simulink model "TriggeredEnabled_Subsystem"  (R2017b)
settings: Solver=FixedStepDiscrete  StartTime=0.0  StopTime=10.0  FixedStep=0.200000  RelTol=1e-3
settings Model: Creator=hbourbou  LastModifiedBy=hbourbou
settings DataIOCC: SaveFormat=StructureWithTime
settings OptimizationCC: LifeSpan=inf
settings DebuggingCC: SFExecutionAtInitializationDiag=none
settings HardwareCC: ProdBitPerSizeT=32  ProdBitPerPtrDiffT=32  ProdWordSize=32  ProdHWDeviceType=Specified
settings CodeAppCC: StateflowObjectComments=on

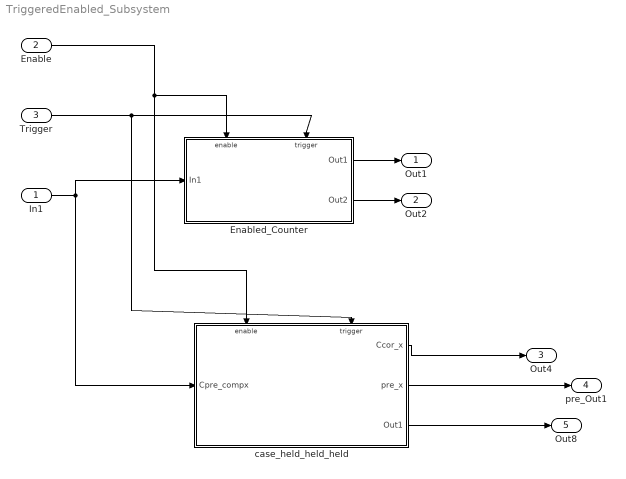
== system TriggeredEnabled_Subsystem ==
  In1 : Inport
  Enable : Inport  Port=2
  Trigger : Inport  Port=3
  Enabled_Counter : Subsystem  TreatAsAtomicUnit=on
  case_held_held_held : Subsystem  TreatAsAtomicUnit=on
  Out1 : Outport
  Out2 : Outport  Port=2
  Out4 : Outport  Port=3
  pre_Out1 : Outport  Port=4
  Out8 : Outport  Port=5
  wires:
  Enabled_Counter/1(Out1) -> Out1/1
  Enabled_Counter/2(Out2) -> Out2/1
  Enable/1 -> case_held_held_held/Enable, Enabled_Counter/Enable
  case_held_held_held/1(Ccor_x) -> Out4/1
  In1/1 -> Enabled_Counter/1(In1), case_held_held_held/1(Cpre_compx)
  case_held_held_held/2(pre_x) -> pre_Out1/1
  case_held_held_held/3(Out1) -> Out8/1
  Trigger/1 -> Enabled_Counter/Trigger, case_held_held_held/Trigger

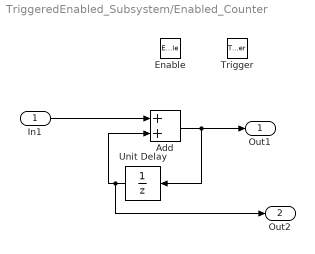
== system TriggeredEnabled_Subsystem/Enabled_Counter ==
  In1 : Inport
  Enable : EnablePort
  Trigger : TriggerPort  VariantControl=(inherit)  PortDimensions=1
  Add : Sum
  Unit Delay : UnitDelay  SampleTime=-1
  Out1 : Outport  InitialOutput=0
  Out2 : Outport  Port=2
  wires:
  Unit Delay/1 -> Out2/1, Add/2
  In1/1 -> Add/1
  Add/1 -> Unit Delay/1, Out1/1

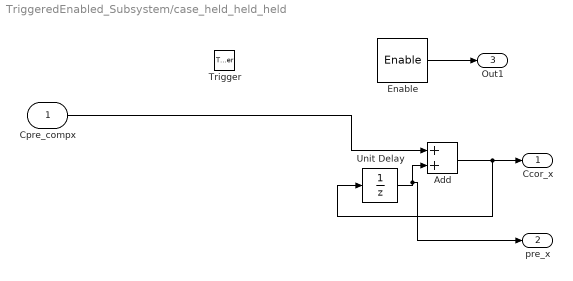
== system TriggeredEnabled_Subsystem/case_held_held_held ==
  Cpre_compx : Inport  OutDataTypeStr=double  PortDimensions=[1]
  Enable : EnablePort  ShowOutputPort=on
  Trigger : TriggerPort  VariantControl=(inherit)  PortDimensions=1
  Add : Sum
  Unit Delay : UnitDelay  SampleTime=-1.0000000000000000
  Ccor_x : Outport  InitialOutput=0
  pre_x : Outport  Port=2  InitialOutput=0
  Out1 : Outport  Port=3
  wires:
  Cpre_compx/1 -> Add/1
  Unit Delay/1 -> pre_x/1, Add/2
  Add/1 -> Unit Delay/1, Ccor_x/1
  Enable/1 -> Out1/1
